simulink model "Rodriguez20213058 [Simulink Hiper]"  (R2023a)
settings: Solver=ode15s  StartTime=0.0  StopTime=10  MaxStep=1e-3  RelTol=1e-3
libraries: slpidlib x1
settings Model: Creator=DELL  LastModifiedBy=biom3
settings DataIOCC: ReturnWorkspaceOutputs=off  TimeSaveName=t
settings DebuggingCC: AlgebraicLoopMsg=none  ArtificialAlgebraicLoopMsg=none  MaxConsecutiveZCsMsg=none  ModelReferenceExtraNoncontSigs=none  OperatingPointInterfaceChecksumMismatchMsg=none

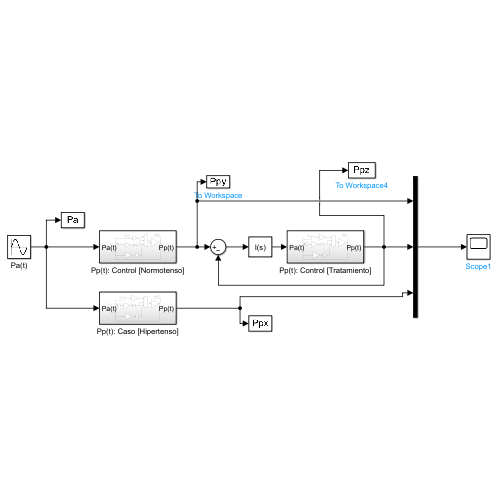
[thumbnail: Simulink's stored preview of the top-level diagram]
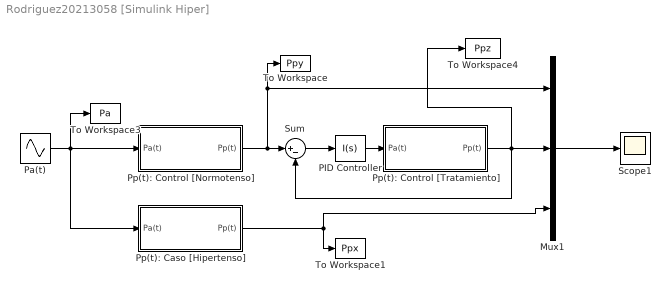
== system Rodriguez20213058 [Simulink Hiper] ==
  Mux1 : Mux  Inputs=3
  PID Controller : slpidlib/PID Controller  Controller=I  Form=Parallel  TimeDomain=Continuous-time  UseExternalTs=off  SampleTime=-1  IntegratorMethod=Forward Euler  FilterMethod=Forward Euler  ControllerParametersSource=internal  P=0  I=1034.73647017467  UseKiTs=off  D=0  N=100  UseFilter=on  TunerSelectOption=Transfer Function Based (PID Tuner App)  InitialConditionSource=internal  InitialConditionForIntegrator=0  InitialConditionForFilter=0  DifferentiatorICPrevScaledInput=0  ExternalReset=none  TrackingMode=off  Kt=1  LimitOutput=off  SatLimitsSource=internal  UpperSaturationLimit=inf  LowerSaturationLimit=-inf  LinearizeAsGain=on  AntiWindupMode=none  Kb=1  LimitIntegrator=off  UpperIntegratorSaturationLimit=inf  LowerIntegratorSaturationLimit=-inf  POutMin=[]  POutMax=[]  IOutMin=[]  IOutMax=[]  DOutMin=[]  DOutMax=[]  NOutMin=[]  NOutMax=[]  SumOutMin=[]  SumOutMax=[]  SaturationOutMin=[]  SaturationOutMax=[]  PParamMin=[]  PParamMax=[]  IParamMin=[]  IParamMax=[]  DParamMin=[]  DParamMax=[]  NParamMin=[]  NParamMax=[]  KbParamMin=[]  KbParamMax=[]  KtParamMin=[]  KtParamMax=[]  KbOutMin=[]  KbOutMax=[]  KtOutMin=[]  KtOutMax=[]  IntegratorOutMin=[]  IntegratorOutMax=[]  FilterOutMin=[]  FilterOutMax=[]  SumI1OutMin=[]  SumI1OutMax=[]  SumI2OutMin=[]  SumI2OutMax=[]  SumI3OutMin=[]  SumI3OutMax=[]  SumI4OutMin=[]  SumI4OutMax=[]  SumDOutMin=[]  SumDOutMax=[]  DifferentiatorOutMin=[]  DifferentiatorOutMax=[]  FilterDiffOutCoefMin=[]  FilterDiffOutCoefMax=[]  ReciprocalOutMin=[]  ReciprocalOutMax=[]  SumDenOutMin=[]  SumDenOutMax=[]  SumNumOutMin=[]  SumNumOutMax=[]  DivideOutMin=[]  DivideOutMax=[]  UdiffTsProdOutMin=[]  UdiffTsProdOutMax=[]  NTsProdOutMin=[]  NTsProdOutMax=[]  UintegralTsProdOutMin=[]  UintegralTsProdOutMax=[]  UngainTsProdOutMin=[]  UngainTsProdOutMax=[]  ClampingZeroOutDataTypeStr=Inherit: Inherit via back propagation  ClampingZeroOutMin=[]  ClampingZeroOutMax=[]  FilterDenConstantOutDataTypeStr=Inherit: Inherit via back propagation  FilterDenConstantOutMin=[]  FilterDenConstantOutMax=[]  PCopyOutDataTypeStr=Inherit: Inherit via back propagation  PCopyOutMin=[]  PCopyOutMax=[]  NCopyOutDataTypeStr=Inherit: Inherit via back propagation  NCopyOutMin=[]  NCopyOutMax=[]  IntegratorContinuousStateAttributes=''  IntegratorStateMustResolveToSignalObject=off  IntegratorRTWStateStorageClass=Auto  FilterContinuousStateAttributes=''  FilterStateMustResolveToSignalObject=off  FilterRTWStateStorageClass=Auto  ParallelPVariant=Disabled  IdealPVariant=Disabled  IVariant=InternalParameters  DVariant=Disabled  IntegratorVariant=Continuous  SatVariant=Disabled  AWVariant=Passthrough  PCopyVariant=Disabled  TRVariant=Disabled  FdbkBlocksVariant=Forward  IdealPFdbkVariant=Disabled  SatFdbkVariant=Disabled  DerivativeFilterVariant=Disabled  NVariant=Disabled  NCopyVariant=Disabled_SignalSpec  FilterICVariant=Disabled  IntegratorICVariant=InternalICs  ExternalResetVariant=Disabled  TRSumVariant=Passthrough  SumFdbkVariant=Disabled  SumVariant=Passthrough_I  TsampFilterVariant=InternalTs  TsampNgainVariant=Passthrough  TsampIntegralVariant=Disabled_SignalSpec  ExternalSaturationOutDataTypeStr=Inherit: Same as second input
  Pa(t) : Sin  Bias=0.8  Frequency=2*pi*95/60  SampleTime=0
  Pp(t): Caso [Hipertenso] : Subsystem
  Pp(t): Control [Normotenso] : Subsystem
  Pp(t): Control [Tratamiento] : Subsystem
  Scope1 : Scope
  Sum : Sum  Inputs=|+-
  To Workspace : ToWorkspace  VariableName=Ppy  SaveFormat=Timeseries  SampleTime=-1
  To Workspace1 : ToWorkspace  VariableName=Ppx  SaveFormat=Timeseries  SampleTime=-1
  To Workspace3 : ToWorkspace  VariableName=Pa  SaveFormat=Timeseries  SampleTime=-1
  To Workspace4 : ToWorkspace  VariableName=Ppz  SaveFormat=Timeseries  SampleTime=-1
  wires:
  PID Controller/1 -> Pp(t): Control [Tratamiento]/1(Pa(t))
  Sum/1 -> PID Controller/1
  Mux1/1 -> Scope1/1
  Pp(t): Control [Normotenso]/1(Pp(t)) -> Mux1/1, To Workspace/1, Sum/1
  Pa(t)/1 -> Pp(t): Caso [Hipertenso]/1(Pa(t)), To Workspace3/1, Pp(t): Control [Normotenso]/1(Pa(t))
  Pp(t): Caso [Hipertenso]/1(Pp(t)) -> Mux1/3, To Workspace1/1
  Pp(t): Control [Tratamiento]/1(Pp(t)) -> To Workspace4/1, Sum/2, Mux1/2

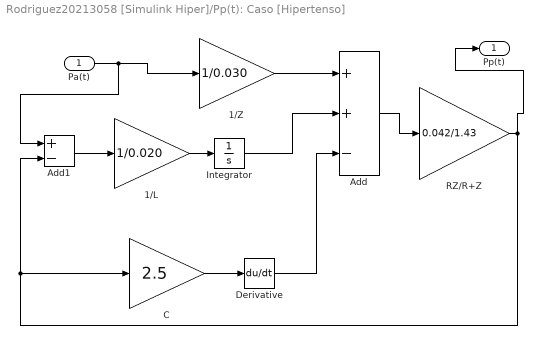
== system Rodriguez20213058 [Simulink Hiper]/Pp(t): Caso [Hipertenso] ==
  Pa(t) : Inport
  1/L : Gain  Gain=1/0.020
  1/Z : Gain  Gain=1/0.030
  Add : Sum  Inputs=++-
  Add1 : Sum  Inputs=+-
  C : Gain  Gain=2.5
  Derivative : Derivative
  Integrator : Integrator
  RZ/R+Z : Gain  Gain=0.042/1.43
  Pp(t) : Outport
  wires:
  1/Z/1 -> Add/1
  Integrator/1 -> Add/2
  C/1 -> Derivative/1
  RZ/R+Z/1 -> Pp(t)/1, Add1/2, C/1
  Add1/1 -> 1/L/1
  Derivative/1 -> Add/3
  1/L/1 -> Integrator/1
  Pa(t)/1 -> Add1/1, 1/Z/1
  Add/1 -> RZ/R+Z/1

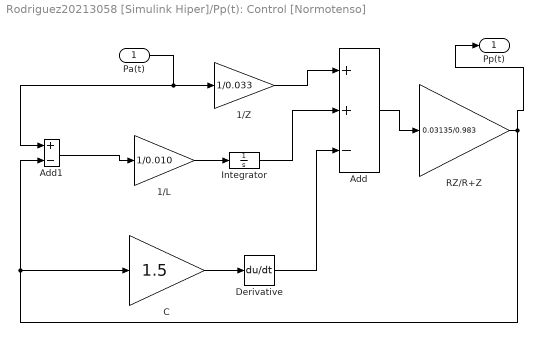
== system Rodriguez20213058 [Simulink Hiper]/Pp(t): Control [Normotenso] ==
  Pa(t) : Inport
  1/L : Gain  Gain=1/0.010
  1/Z : Gain  Gain=1/0.033
  Add : Sum  Inputs=++-
  Add1 : Sum  Inputs=+-
  C : Gain  Gain=1.5
  Derivative : Derivative
  Integrator : Integrator
  RZ/R+Z : Gain  Gain=0.03135/0.983
  Pp(t) : Outport
  wires:
  Pa(t)/1 -> Add1/1, 1/Z/1
  1/Z/1 -> Add/1
  Integrator/1 -> Add/2
  1/L/1 -> Integrator/1
  Add1/1 -> 1/L/1
  Add/1 -> RZ/R+Z/1
  C/1 -> Derivative/1
  Derivative/1 -> Add/3
  RZ/R+Z/1 -> Pp(t)/1, Add1/2, C/1

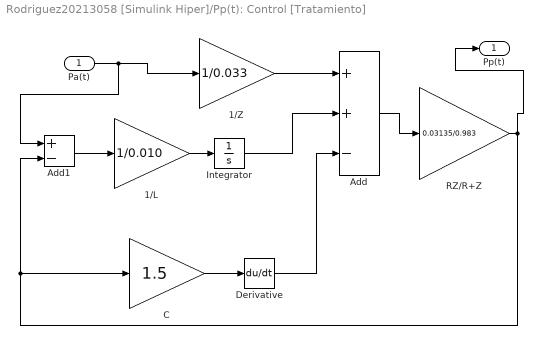
== system Rodriguez20213058 [Simulink Hiper]/Pp(t): Control [Tratamiento] ==
  Pa(t) : Inport
  1/L : Gain  Gain=1/0.010
  1/Z : Gain  Gain=1/0.033
  Add : Sum  Inputs=++-
  Add1 : Sum  Inputs=+-
  C : Gain  Gain=1.5
  Derivative : Derivative
  Integrator : Integrator
  RZ/R+Z : Gain  Gain=0.03135/0.983
  Pp(t) : Outport
  wires:
  1/Z/1 -> Add/1
  Integrator/1 -> Add/2
  C/1 -> Derivative/1
  RZ/R+Z/1 -> Pp(t)/1, Add1/2, C/1
  Add1/1 -> 1/L/1
  Derivative/1 -> Add/3
  1/L/1 -> Integrator/1
  Pa(t)/1 -> Add1/1, 1/Z/1
  Add/1 -> RZ/R+Z/1
